simulink model "power_rectifier"  (Simulink 6.0)
settings: Solver=ode23tb  SolverMode=SingleTasking  StartTime=0.0  StopTime=0.1  RelTol=1e-3
libraries: powerlib x19
settings Model: Creator=patrice  LastModifiedBy=batserve  ExtModeTrigMode=oneshot  ExtModeArmWhenConnect=off  ExtModeAutoUpdateStatusClock=off
settings DataIOCC: LimitDataPoints=off  SignalLoggingName=sigsOut
settings OptimizationCC: BlockReduction=off  BooleanDataType=off
settings DebuggingCC: CheckExecutionContextPreStartOutputMsg=on  CheckExecutionContextRuntimeOutputMsg=on  SolverPrmCheckMsg=none
settings HardwareCC: TargetUnknown=on
settings RTWCC: TemplateMakefile=grt_unix.tmf

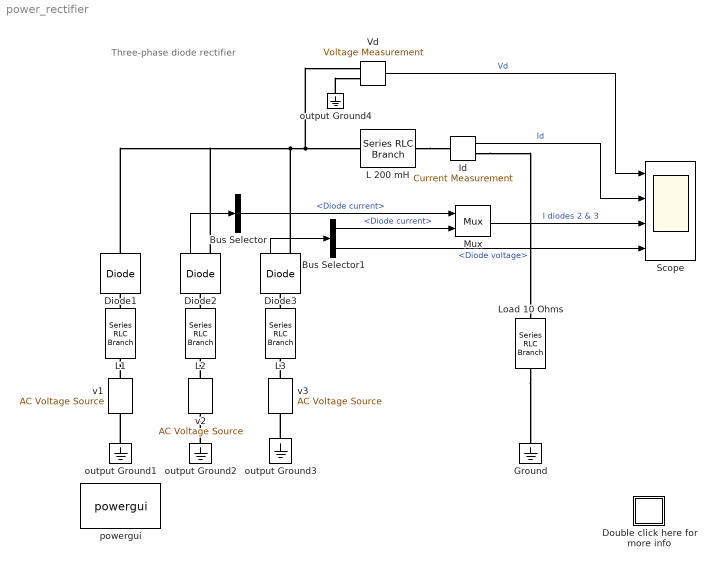
== system power_rectifier ==
  note: Three-phase diode rectifier
  Bus Selector : BusSelector  DialogController=Simulink.DDGSource_Bus  OutputSignals=Diode current
  Bus Selector1 : BusSelector  DialogController=Simulink.DDGSource_Bus  OutputSignals=Diode current,Diode voltage
  Diode1 : powerlib/Power Electronics/Diode  Orientation=up  Ron=1e-2  Lon=0  Vf=0.8  IC=0  Rs=1000  Cs=0.1e-6  Measurements=off
  Diode2 : powerlib/Power Electronics/Diode  Orientation=up  Ron=1e-2  Lon=0  Vf=0.8  IC=0  Rs=1000  Cs=0.1e-6  Measurements=on
  Diode3 : powerlib/Power Electronics/Diode  Orientation=up  Ron=1e-2  Lon=0  Vf=0.8  IC=0  Rs=1000  Cs=0.1e-6  Measurements=on
  Double click here for more info : Subsystem
      mask Display: disp('?')
  Ground : powerlib/Elements/Ground  Orientation=down  PhysicalDomain=powersysdomain  SubClassName=unknown  LeftPortType=p1  RightPortType=p1  LConnTagsString=a
  Id : powerlib/Measurements/Current Measurement  Tag=PoWeRsYsTeMmEaSuReMeNt  PhasorSimulation=off  OutputType=Magnitude  PSBequivalent=0
  L 200 mH : powerlib/Elements/Series RLC Branch  PhysicalDomain=powersysdomain  SubClassName=unknown  LeftPortType=p1  RightPortType=p1  LConnTagsString=__new0  RConnTagsString=__new0  Resistance=0  Inductance=200e-03  Capacitance=inf  Measurements=None
  L1 : powerlib/Elements/Series RLC Branch  Orientation=up  PhysicalDomain=powersysdomain  SubClassName=unknown  LeftPortType=p1  RightPortType=p1  LConnTagsString=__new0  RConnTagsString=__new0  Resistance=0  Inductance=5e-03  Capacitance=inf  Measurements=None
  L2 : powerlib/Elements/Series RLC Branch  Orientation=up  PhysicalDomain=powersysdomain  SubClassName=unknown  LeftPortType=p1  RightPortType=p1  LConnTagsString=__new0  RConnTagsString=__new0  Resistance=0  Inductance=5e-03  Capacitance=inf  Measurements=None
  L3 : powerlib/Elements/Series RLC Branch  Orientation=up  PhysicalDomain=powersysdomain  SubClassName=unknown  LeftPortType=p1  RightPortType=p1  LConnTagsString=__new0  RConnTagsString=__new0  Resistance=0  Inductance=5e-03  Capacitance=inf  Measurements=None
  Load 10 Ohms : powerlib/Elements/Series RLC Branch  Orientation=down  PhysicalDomain=powersysdomain  SubClassName=unknown  LeftPortType=p1  RightPortType=p1  LConnTagsString=__new0  RConnTagsString=__new0  Resistance=10  Inductance=0  Capacitance=inf  Measurements=None
  Mux : Mux  Inputs=2
  Scope : Scope  NumInputPorts=4
      settings: TimeRange=0.1  YMin=0~0~0~-500  YMax=200~20~20~500  DataFormat=Structure
  Vd : powerlib/Measurements/Voltage Measurement  Tag=PoWeRsYsTeMmEaSuReMeNt  PhasorSimulation=off  OutputType=Magnitude  PSBequivalent=0
  output Ground{1..4} (4 alike) : powerlib/Elements/Ground  Orientation=down  PhysicalDomain=powersysdomain  SubClassName=unknown  LeftPortType=p1  RightPortType=p1  LConnTagsString=a
  powergui : powerlib/powergui  Priority=2  Frange=[0:2:500]  Ylog=off  Xlog=on  save=off  variable=ZData  ZoomFFT=on  StartTime=0.0  cycles=1  DisplayStyle=1  fundamental=60  FreqAxis=off  MaxFrequency=1000  frequencyindice=1  frequencyindicesteady=1  RmsSteady=1  display=off  Ts=0  methode=off  frequency=60  echomessages=on
  v1 : powerlib/Electrical Sources/AC Voltage Source  Description=source block  Orientation=up  Amplitude=120*sqrt(2)  Phase=0  Frequency=60  SampleTime=0  Measurements=None
      settings: AttributesFormatString=\n
  v2 : powerlib/Electrical Sources/AC Voltage Source  Description=source block  Orientation=up  Amplitude=120*sqrt(2)  Phase=-120  Frequency=60  SampleTime=0  Measurements=None
      settings: AttributesFormatString=\n
  v3 : powerlib/Electrical Sources/AC Voltage Source  Description=source block  Orientation=up  Amplitude=120*sqrt(2)  Phase=120  Frequency=60  SampleTime=0  Measurements=None
      settings: AttributesFormatString=\n
  wires:
  Bus Selector1/1 -> Mux/2  "<Diode current>"
  Mux/1 -> Scope/3  "I diodes 2 & 3"
  Bus Selector1/2 -> Scope/4  "<Diode voltage>"
  Diode2/1 -> Bus Selector/1
  Vd/1 -> Scope/1  "Vd"
  Id/1 -> Scope/2  "Id"
  Diode3/1 -> Bus Selector1/1
  Bus Selector/1 -> Mux/1  "<Diode current>"
  connections:
  L 200 mH/RConn1 -- Id/LConn1
  Id/RConn1 -- Load 10 Ohms/LConn1
  Load 10 Ohms/RConn1 -- Ground/LConn1
  output Ground1/LConn1 -- v1/LConn1
  L1/RConn1 -- Diode1/LConn1
  v1/RConn1 -- L1/LConn1
  output Ground2/LConn1 -- v2/LConn1
  L2/RConn1 -- Diode2/LConn1
  v2/RConn1 -- L2/LConn1
  output Ground3/LConn1 -- v3/LConn1
  L3/RConn1 -- Diode3/LConn1
  v3/RConn1 -- L3/LConn1
  Diode1/RConn1 -- Diode2/RConn1 -- L 200 mH/LConn1 -- Vd/LConn1 -- Diode3/RConn1
  output Ground4/LConn1 -- Vd/LConn2

== system power_rectifier/Double click here for more info ==
  note: Demonstration
  note: Description
  note: This demonstration illustrates use of the Diode block
      | to simulate a three-phase rectifier and
      | compares continuous vs discrete simulations
  note: A 10 ohm load is fed in DC through a three-phase rectifier from an inductive
      | source (5 mH; 120 V rms). The rectified current is filtered by a 200mH inductance.
      |
      | Diodes are connected in parallel with RC snubbers (1000 ohms-0.1 uF)
      | The measurement outputs of Diode2 and  Diode3 is used to observe the diode voltage and current.
  note: 1. Simulation with continuous integration method
  note: 2. Simulation with discretized system
  note: Open the Powergui block menu. select 'Discretize electrical model' and specify a sample time of 50e-6 secs.
      | Restart the simulation.
      |
      | Your system is now discretized and simulated at fixed time steps.
      | Compare  waveforms with those obtained with the continuous integration algorithm (ode23tb).
  note: G. Sybille (Hydro-Quebec)
  note: Check  the simulation parameters in the Simulation/Parameters menu
      | The following intregation algorithm should be used: Variable time step ode23tb with default parameters.
      | Start the simulation and observe waveforms on the four trace Scope block.
      |
      | After a transient period the load current Id stabilizes at  12.7 A.  Note that  most of the  third harmonic which
      | can be seen in the rectified voltage Vd  (mean value 127 V) is filtered out by the  smoothing reactor.
      |
      | Observe also the commutation period due to the source inductances.
      | The 3.3 degrees  overlap is clearly seen on  trace 3 of  the scope showing currents in  diodes 2 and 3.
      |
      | Zoom on the Diode3 voltage (trace 4) during the conduction period. The voltage magnitude is the sum of the
      | specified  forward voltage (0.8 V) and the voltage developed  across the diode resistance (0.01 ohm).
